simulink library "SimscapeFPGAHIL_lib"  (R2023b)
settings: Solver=VariableStepAuto  StartTime=0.0  StopTime=10.0  RelTol=1e-3
undefined symbols (not defined in the file): a, b, c, DiscIntNeverNeededParam, threshold
libraries: fl_lib x16, nesl_utility x12, simulink x10, fpga_utils_lib x4, hdlsllib x2, $bdroot x1
settings Model: Creator=The MathWorks, Inc.  LastModifiedBy=promero

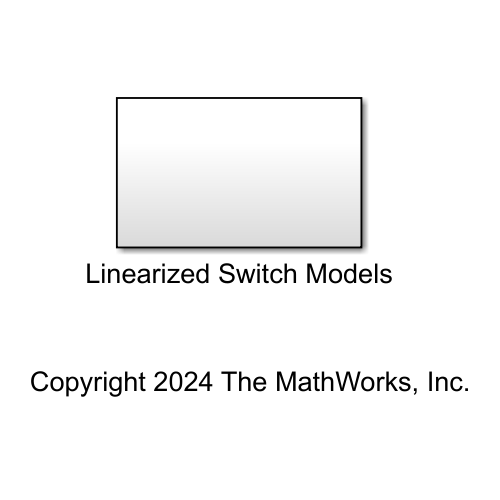
[thumbnail: Simulink's stored preview of the top-level diagram]
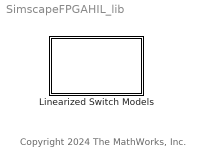
== system SimscapeFPGAHIL_lib ==
  note: Copyright 2024 The MathWorks, Inc.
  Linearized Switch Models : Subsystem

== system SimscapeFPGAHIL_lib/Linearized Switch Models ==
  note: Linear time-invariant approximation of piecewise linear switching elements
  Diode : Subsystem  mask{Vf=0.6, Gs=1, s=1}
      mask prompts: Vf "Forward voltage [V]"; Gs "Conductance (1/Ohm)"; s "Time scaling"
      settings: CopyFcn=set_param(gcb, 'LinkStatus', 'none');
      mask TypeOptions Vf: Controller/Vf
      mask TypeOptions s: Controller/s
  IGBT : Subsystem  mask{Vth=0.5, Vf=0.8, Gs=1, s=1, avgFactor=1, isFixedPoint=off}
      mask prompts: Vth "Threshold voltage [V]"; Vf "Forward voltage [V]"; Gs "Conductance [1/Ohm]"; s "Time scaling"; avgFactor "Subcycle average factor"; isFixedPoint "Use fixed point for Subcycle Average"
      settings: CopyFcn=set_param(gcb, 'LinkStatus', 'none');
      mask TypeOptions Vth: Controller/Vth
      mask TypeOptions Vf: Controller/Vf
      mask TypeOptions s: Controller/s
      mask TypeOptions avgFactor: Controller/avgFactor
      mask TypeOptions isFixedPoint: Controller/isFixedPoint
  MOSFET : Subsystem  mask{threshold=0.5, Gs=1, s=1, avgFactor=1, isFixedPoint=off}
      mask prompts: threshold "Threshold voltage [V]"; Gs "Conductance (1/Ohm)"; s "Time scaling"; avgFactor "Subcycle average factor"; isFixedPoint "Use fixed-point for Subcycle Average"
      settings: CopyFcn=set_param(gcb, 'LinkStatus', 'none');
      mask TypeOptions threshold: Controller/threshold
      mask TypeOptions s: Controller/s
      mask TypeOptions avgFactor: Controller/avgFactor
      mask TypeOptions isFixedPoint: Controller/isFixedPoint
  Switch : Subsystem  mask{threshold=0.5, Gs=1, s=1, avgFactor=1, isFixedPoint=off}
      mask prompts: threshold "Threshold voltage [V]"; Gs "Conductance (1/Ohm)"; s "Time scaling"; avgFactor "Subcycle average factor"; isFixedPoint "Use fixed-point for Subcycle Average"
      settings: CopyFcn=set_param(gcb, 'LinkStatus', 'none');
      mask TypeOptions threshold: Controller/threshold
      mask TypeOptions s: Controller/s
      mask TypeOptions avgFactor: Controller/avgFactor
      mask TypeOptions isFixedPoint: Controller/isFixedPoint

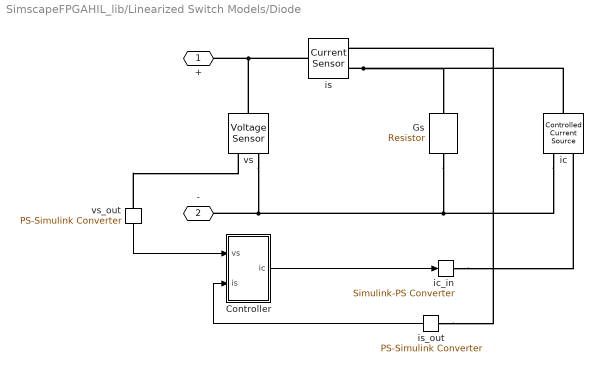
== system SimscapeFPGAHIL_lib/Linearized Switch Models/Diode ==
  Controller : Subsystem  mask{Vf=Vf, Gs=Gs, s=s}
      mask prompts: Vf "Forward voltage [V]"; Gs "Conductance [1/Ohm]"; s "Time scaling"
      mask DialogControl DescGroupVar Prompt: Description
      mask DialogControl Details Prompt: Diode Controller
  Gs : fl_lib/Electrical/Electrical Elements/Resistor  R=1/Gs Ohm  i_specify=off  i_priority=None  i=0 A  i_nominal_specify=off  i_nominal_unit=A  i_nominal_value=1  v_specify=off  v_priority=None  v=0 V  v_nominal_specify=off  v_nominal_unit=V  v_nominal_value=1
      settings: LibrarySourceBlock=SimscapeFPGAHIL_lib/Linearized Switch Models/Switch/Gs
  ic : fl_lib/Electrical/Electrical Sources/Controlled Current Source
      settings: LibrarySourceBlock=SimscapeFPGAHIL_lib/Linearized Switch Models/Switch/ic
  ic_in : nesl_utility/Simulink-PS Converter  PhysicalDomain=network_engine_domain  SubClassName=ps_input  LeftPortType=input  RightPortType=output  PseudoPeriodic=off  Frequencies=[]  NoiseDistribution=none  NoiseParameters=[]  Unit=A  AffineConversion=off  FilteringAndDerivatives=provide  SimscapeFilterOrder=1  InputFilterTimeConstant=0.001  UdotUserProvided=0
      settings: LibrarySourceBlock=SimscapeFPGAHIL_lib/Linearized Switch Models/Switch/ic_in
  is : fl_lib/Electrical/Electrical Sensors/Current Sensor
      settings: LibrarySourceBlock=SimscapeFPGAHIL_lib/Linearized Switch Models/Switch/is
  is_out : nesl_utility/PS-Simulink Converter  PhysicalDomain=network_engine_domain  SubClassName=ps_output  LeftPortType=input  RightPortType=output  PseudoPeriodic=off  Frequencies=[]  VectorFormat=1-D array  Unit=A  AffineConversion=off
      settings: LibrarySourceBlock=SimscapeFPGAHIL_lib/Linearized Switch Models/Switch/is_out
  vs : fl_lib/Electrical/Electrical Sensors/Voltage Sensor
      settings: LibrarySourceBlock=SimscapeFPGAHIL_lib/Linearized Switch Models/Switch/vs
  vs_out : nesl_utility/PS-Simulink Converter  PhysicalDomain=network_engine_domain  SubClassName=ps_output  LeftPortType=input  RightPortType=output  PseudoPeriodic=off  Frequencies=[]  VectorFormat=1-D array  Unit=V  AffineConversion=off
      settings: LibrarySourceBlock=SimscapeFPGAHIL_lib/Linearized Switch Models/Switch/vs_out
  + : PMIOPort  Side=Left
  - : PMIOPort  Port=2  Side=Right
  wires:
  Controller/1(ic) -> ic_in/1
  is_out/1 -> Controller/2(is)
  vs_out/1 -> Controller/1(vs)
  connections:
  is_out/LConn1 -- is/RConn1
  vs_out/LConn1 -- vs/RConn1
  ic_in/RConn1 -- ic/RConn1
  is/LConn1 -- +/RConn1 -- vs/LConn1
  ic/RConn2 -- Gs/RConn1 -- -/RConn1 -- vs/RConn2
  is/RConn2 -- Gs/LConn1 -- ic/LConn1

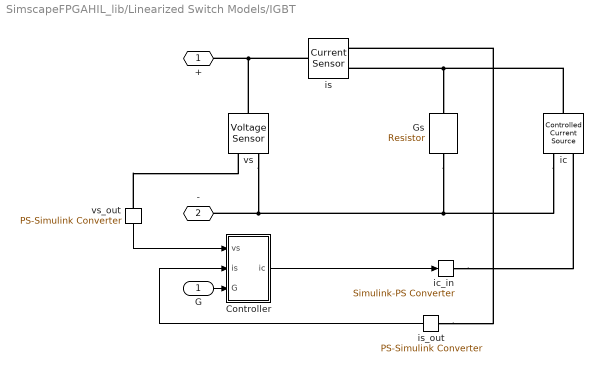
== system SimscapeFPGAHIL_lib/Linearized Switch Models/IGBT ==
  G : Inport
  Controller : Subsystem  mask{Vf=Vf, Vth=Vth, Gs=Gs, s=s, avgFactor=avgFactor, isFixedPoint=off}
      mask prompts: Vf "Forward voltage (V)"; Vth "Threshold voltage (V)"; Gs "Conductance (1/Ohm)"; s "Time scaling"; avgFactor "Subcycle average factor"; isFixedPoint "Use fixed point for Subcycle Average"
      mask DialogControl DescGroupVar Prompt: Description
      mask DialogControl Details Prompt: IGBT Controller
  Gs : fl_lib/Electrical/Electrical Elements/Resistor  R=1/Gs Ohm  i_specify=off  i_priority=None  i=0 A  i_nominal_specify=off  i_nominal_unit=A  i_nominal_value=1  v_specify=off  v_priority=None  v=0 V  v_nominal_specify=off  v_nominal_unit=V  v_nominal_value=1
      settings: LibrarySourceBlock=SimscapeFPGAHIL_lib/Linearized Switch Models/MOSFET/Gs
  ic : fl_lib/Electrical/Electrical Sources/Controlled Current Source
      settings: LibrarySourceBlock=SimscapeFPGAHIL_lib/Linearized Switch Models/MOSFET/ic
  ic_in : nesl_utility/Simulink-PS Converter  PhysicalDomain=network_engine_domain  SubClassName=ps_input  LeftPortType=input  RightPortType=output  PseudoPeriodic=off  Frequencies=[]  NoiseDistribution=none  NoiseParameters=[]  Unit=A  AffineConversion=off  FilteringAndDerivatives=provide  SimscapeFilterOrder=1  InputFilterTimeConstant=0.001  UdotUserProvided=0
      settings: LibrarySourceBlock=SimscapeFPGAHIL_lib/Linearized Switch Models/MOSFET/ic_in
  is : fl_lib/Electrical/Electrical Sensors/Current Sensor
      settings: LibrarySourceBlock=SimscapeFPGAHIL_lib/Linearized Switch Models/MOSFET/is
  is_out : nesl_utility/PS-Simulink Converter  PhysicalDomain=network_engine_domain  SubClassName=ps_output  LeftPortType=input  RightPortType=output  PseudoPeriodic=off  Frequencies=[]  VectorFormat=1-D array  Unit=A  AffineConversion=off
      settings: LibrarySourceBlock=SimscapeFPGAHIL_lib/Linearized Switch Models/MOSFET/is_out
  vs : fl_lib/Electrical/Electrical Sensors/Voltage Sensor
      settings: LibrarySourceBlock=SimscapeFPGAHIL_lib/Linearized Switch Models/MOSFET/vs
  vs_out : nesl_utility/PS-Simulink Converter  PhysicalDomain=network_engine_domain  SubClassName=ps_output  LeftPortType=input  RightPortType=output  PseudoPeriodic=off  Frequencies=[]  VectorFormat=1-D array  Unit=V  AffineConversion=off
      settings: LibrarySourceBlock=SimscapeFPGAHIL_lib/Linearized Switch Models/MOSFET/vs_out
  + : PMIOPort  Side=Left
  - : PMIOPort  Port=2  Side=Right
  wires:
  vs_out/1 -> Controller/1(vs)
  is_out/1 -> Controller/2(is)
  G/1 -> Controller/3(G)
  Controller/1(ic) -> ic_in/1
  connections:
  ic/LConn1 -- Gs/LConn1 -- is/RConn2
  vs/RConn2 -- -/RConn1 -- Gs/RConn1 -- ic/RConn2
  vs/LConn1 -- +/RConn1 -- is/LConn1
  ic_in/RConn1 -- ic/RConn1
  vs_out/LConn1 -- vs/RConn1
  is_out/LConn1 -- is/RConn1

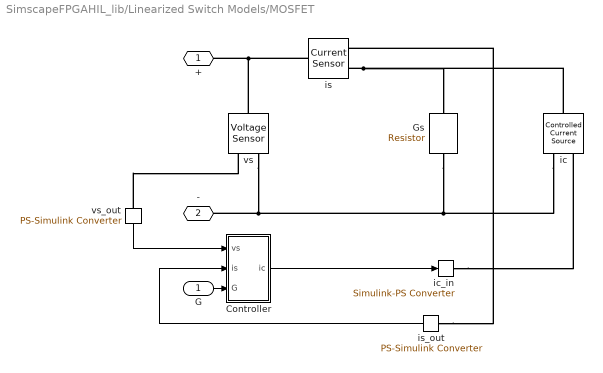
== system SimscapeFPGAHIL_lib/Linearized Switch Models/MOSFET ==
  G : Inport
  Controller : Subsystem  mask{threshold=threshold, Gs=Gs, s=s, avgFactor=avgFactor, isFixedPoint=off}
      mask prompts: threshold "Threshold voltage [V]"; Gs "Conductance (1/Ohm)"; s "Time scaling"; avgFactor "Subcycle average factor"; isFixedPoint "Use fixed-point for Subcycle Average"
      mask DialogControl DescGroupVar Prompt: Description
      mask DialogControl Details Prompt: Switch Controller
  Gs : fl_lib/Electrical/Electrical Elements/Resistor  R=1/Gs Ohm  i_specify=off  i_priority=None  i=0 A  i_nominal_specify=off  i_nominal_unit=A  i_nominal_value=1  v_specify=off  v_priority=None  v=0 V  v_nominal_specify=off  v_nominal_unit=V  v_nominal_value=1
  ic : fl_lib/Electrical/Electrical Sources/Controlled Current Source
  ic_in : nesl_utility/Simulink-PS Converter  PhysicalDomain=network_engine_domain  SubClassName=ps_input  LeftPortType=input  RightPortType=output  PseudoPeriodic=off  Frequencies=[]  NoiseDistribution=none  NoiseParameters=[]  Unit=A  AffineConversion=off  FilteringAndDerivatives=provide  SimscapeFilterOrder=1  InputFilterTimeConstant=0.001  UdotUserProvided=0
  is : fl_lib/Electrical/Electrical Sensors/Current Sensor
  is_out : nesl_utility/PS-Simulink Converter  PhysicalDomain=network_engine_domain  SubClassName=ps_output  LeftPortType=input  RightPortType=output  PseudoPeriodic=off  Frequencies=[]  VectorFormat=1-D array  Unit=A  AffineConversion=off
  vs : fl_lib/Electrical/Electrical Sensors/Voltage Sensor
  vs_out : nesl_utility/PS-Simulink Converter  PhysicalDomain=network_engine_domain  SubClassName=ps_output  LeftPortType=input  RightPortType=output  PseudoPeriodic=off  Frequencies=[]  VectorFormat=1-D array  Unit=V  AffineConversion=off
  + : PMIOPort  Side=Left
  - : PMIOPort  Port=2  Side=Right
  wires:
  Controller/1(ic) -> ic_in/1
  G/1 -> Controller/3(G)
  is_out/1 -> Controller/2(is)
  vs_out/1 -> Controller/1(vs)
  connections:
  is_out/LConn1 -- is/RConn1
  vs_out/LConn1 -- vs/RConn1
  ic_in/RConn1 -- ic/RConn1
  is/LConn1 -- +/RConn1 -- vs/LConn1
  ic/RConn2 -- Gs/RConn1 -- -/RConn1 -- vs/RConn2
  is/RConn2 -- Gs/LConn1 -- ic/LConn1

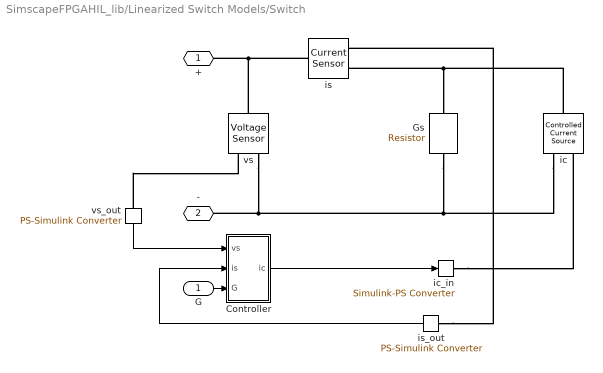
== system SimscapeFPGAHIL_lib/Linearized Switch Models/Switch ==
  G : Inport
  Controller : Subsystem  mask{threshold=threshold, Gs=Gs, s=s, avgFactor=avgFactor, isFixedPoint=off}
      mask prompts: threshold "Threshold voltage [V]"; Gs "Conductance (1/Ohm)"; s "Time scaling"; avgFactor "Subcycle average factor"; isFixedPoint "Use fixed-point for Subcycle Average"
      mask DialogControl DescGroupVar Prompt: Description
      mask DialogControl Details Prompt: Switch Controller
  Gs : fl_lib/Electrical/Electrical Elements/Resistor  R=1/Gs Ohm  i_specify=off  i_priority=None  i=0 A  i_nominal_specify=off  i_nominal_unit=A  i_nominal_value=1  v_specify=off  v_priority=None  v=0 V  v_nominal_specify=off  v_nominal_unit=V  v_nominal_value=1
  ic : fl_lib/Electrical/Electrical Sources/Controlled Current Source
  ic_in : nesl_utility/Simulink-PS Converter  PhysicalDomain=network_engine_domain  SubClassName=ps_input  LeftPortType=input  RightPortType=output  PseudoPeriodic=off  Frequencies=[]  NoiseDistribution=none  NoiseParameters=[]  Unit=A  AffineConversion=off  FilteringAndDerivatives=provide  SimscapeFilterOrder=1  InputFilterTimeConstant=0.001  UdotUserProvided=0
  is : fl_lib/Electrical/Electrical Sensors/Current Sensor
  is_out : nesl_utility/PS-Simulink Converter  PhysicalDomain=network_engine_domain  SubClassName=ps_output  LeftPortType=input  RightPortType=output  PseudoPeriodic=off  Frequencies=[]  VectorFormat=1-D array  Unit=A  AffineConversion=off
  vs : fl_lib/Electrical/Electrical Sensors/Voltage Sensor
  vs_out : nesl_utility/PS-Simulink Converter  PhysicalDomain=network_engine_domain  SubClassName=ps_output  LeftPortType=input  RightPortType=output  PseudoPeriodic=off  Frequencies=[]  VectorFormat=1-D array  Unit=V  AffineConversion=off
  + : PMIOPort  Side=Left
  - : PMIOPort  Port=2  Side=Right
  wires:
  vs_out/1 -> Controller/1(vs)
  is_out/1 -> Controller/2(is)
  G/1 -> Controller/3(G)
  Controller/1(ic) -> ic_in/1
  connections:
  ic/LConn1 -- Gs/LConn1 -- is/RConn2
  vs/RConn2 -- -/RConn1 -- Gs/RConn1 -- ic/RConn2
  vs/LConn1 -- +/RConn1 -- is/LConn1
  ic_in/RConn1 -- ic/RConn1
  vs_out/LConn1 -- vs/RConn1
  is_out/LConn1 -- is/RConn1

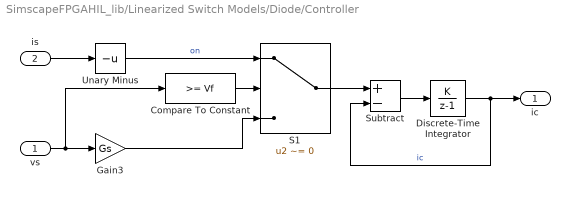
== system SimscapeFPGAHIL_lib/Linearized Switch Models/Diode/Controller ==
  vs : Inport
  is : Inport  Port=2
  Compare To Constant : simulink/Logic and Bit Operations/Compare To Constant  relop=>=  const=Vf  OutDataTypeStr=boolean
      settings: LibrarySourceBlock=|
      | SimscapeFPGAHIL_lib/Linearized Switch Models/Switch/Controller/Switch State/Switch/Compare
      | To Constant
  Discrete-Time Integrator : DiscreteIntegrator  IntegratorMethod=Accumulation: Forward Euler  gainval=1/s  SampleTime=-1  OutDataTypeStr=Inherit: Inherit via back propagation  ICPrevOutput=DiscIntNeverNeededParam  ICPrevScaledInput=DiscIntNeverNeededParam
  Gain3 : Gain  Gain=Gs  OutDataTypeStr=Inherit: Inherit via back propagation
  S1 : Switch  Criteria=u2 ~= 0  Threshold=threshold  SaturateOnIntegerOverflow=off
  Subtract : Sum  Inputs=+-
  Unary Minus : UnaryMinus
  ic : Outport
  wires:
  vs/1 -> Compare To Constant/1, Gain3/1
  is/1 -> Unary Minus/1
  Discrete-Time Integrator/1 -> ic/1, Subtract/2  "ic"
  Subtract/1 -> Discrete-Time Integrator/1
  Gain3/1 -> S1/3
  Unary Minus/1 -> S1/1  "on"
  Compare To Constant/1 -> S1/2
  S1/1 -> Subtract/1

== system SimscapeFPGAHIL_lib/Linearized Switch Models/IGBT/Controller ==
  vs : Inport
  is : Inport  Port=2
  G : Inport  Port=3
  Discrete-Time Integrator : DiscreteIntegrator  IntegratorMethod=Accumulation: Forward Euler  gainval=1/s  SampleTime=-1  OutDataTypeStr=Inherit: Inherit via back propagation  ICPrevOutput=DiscIntNeverNeededParam  ICPrevScaledInput=DiscIntNeverNeededParam
  Subtract : Sum  Inputs=+-
  Switch State : Subsystem  Variant=on  VariantControl=Choice
  Unary Minus : UnaryMinus
  ic : Outport
  wires:
  Unary Minus/1 -> Switch State/1(on)  "on"
  Switch State/1(ic) -> Subtract/1
  Subtract/1 -> Discrete-Time Integrator/1
  Discrete-Time Integrator/1 -> Subtract/2, ic/1  "ic"
  is/1 -> Unary Minus/1
  vs/1 -> Switch State/3(vs)
  G/1 -> Switch State/2(G)

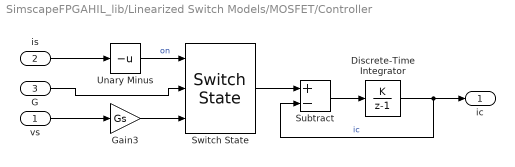
== system SimscapeFPGAHIL_lib/Linearized Switch Models/MOSFET/Controller ==
  vs : Inport
  is : Inport  Port=2
  G : Inport  Port=3
  Discrete-Time Integrator : DiscreteIntegrator  IntegratorMethod=Accumulation: Forward Euler  gainval=1/s  SampleTime=-1  OutDataTypeStr=Inherit: Inherit via back propagation  ICPrevOutput=DiscIntNeverNeededParam  ICPrevScaledInput=DiscIntNeverNeededParam
  Gain3 : Gain  Gain=Gs  OutDataTypeStr=Inherit: Inherit via back propagation
  Subtract : Sum  Inputs=+-
  Switch State : $bdroot/Linearized Switch Models/Switch/Controller/Switch State  SystemSampleTime=-1  VariantControl=Choice  VariantActivationTime=update diagram  AllowFlexibleInterface=on  Latency=0  AutoFrameSizeCalculation=off
      settings: LibrarySourceBlock=SimscapeFPGAHIL_lib/Linearized Switch Models/MOSFET/Controller/Controller/Switch State
  Unary Minus : UnaryMinus
  ic : Outport
  wires:
  Switch State/1 -> Subtract/1
  Gain3/1 -> Switch State/3
  G/1 -> Switch State/2
  Unary Minus/1 -> Switch State/1  "on"
  is/1 -> Unary Minus/1
  Discrete-Time Integrator/1 -> ic/1, Subtract/2  "ic"
  Subtract/1 -> Discrete-Time Integrator/1
  vs/1 -> Gain3/1

== system SimscapeFPGAHIL_lib/Linearized Switch Models/Switch/Controller ==
  vs : Inport
  is : Inport  Port=2
  G : Inport  Port=3
  Discrete-Time Integrator : DiscreteIntegrator  IntegratorMethod=Accumulation: Forward Euler  gainval=1/s  SampleTime=-1  OutDataTypeStr=Inherit: Inherit via back propagation  ICPrevOutput=DiscIntNeverNeededParam  ICPrevScaledInput=DiscIntNeverNeededParam
  Gain3 : Gain  Gain=Gs  OutDataTypeStr=Inherit: Inherit via back propagation
  Subtract : Sum  Inputs=+-
  Switch State : Subsystem  Variant=on  VariantControl=Choice
  Unary Minus : UnaryMinus
  ic : Outport
  wires:
  vs/1 -> Gain3/1
  Subtract/1 -> Discrete-Time Integrator/1
  Discrete-Time Integrator/1 -> ic/1, Subtract/2  "ic"
  is/1 -> Unary Minus/1
  Unary Minus/1 -> Switch State/1(on)  "on"
  G/1 -> Switch State/2(G)
  Gain3/1 -> Switch State/3(off)
  Switch State/1(ic) -> Subtract/1

== system SimscapeFPGAHIL_lib/Linearized Switch Models/IGBT/Controller/Switch State ==
  on : Inport
  G : Inport  Port=2
  vs : Inport  Port=3
  Subcycle Average (Fixed Point) : Subsystem  VariantControl=avgFactor > 1 && isFixedPoint
      settings: LibrarySourceBlock=SimscapeFPGAHIL_lib/Linearized Switch Models/IGBT/Controller/Switch State/Subcycle Average
  Subcycle Average (Floating Point) : Subsystem  VariantControl=avgFactor > 1 && ~isFixedPoint
  Switch : Subsystem  VariantControl=avgFactor == 1
  ic : Outport

== system SimscapeFPGAHIL_lib/Linearized Switch Models/Switch/Controller/Switch State ==
  on : Inport
  G : Inport  Port=2
  off : Inport  Port=3
  Subcycle Average (Fixed-Point) : Subsystem  VariantControl=avgFactor > 1 && isFixedPoint == true
  Subcycle Average (Floating-Point) : Subsystem  VariantControl=avgFactor > 1 && isFixedPoint == false
  Switch : Subsystem  VariantControl=avgFactor == 1
  ic : Outport

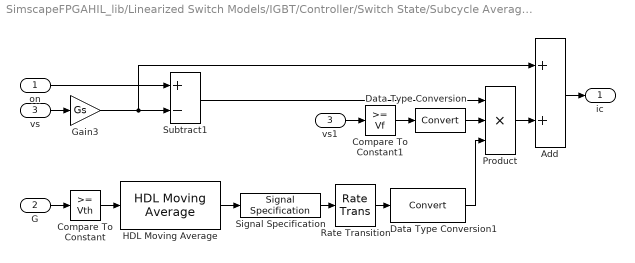
== system SimscapeFPGAHIL_lib/Linearized Switch Models/IGBT/Controller/Switch State/Subcycle Average (Fixed Point) ==
  on : Inport
  G : Inport  Port=2
  vs : Inport  Port=3
  Add : Sum
  Compare To Constant : simulink/Logic and Bit Operations/Compare To Constant  relop=>=  const=Vth  OutDataTypeStr=boolean
      settings: LibrarySourceBlock=|
      | SimscapeFPGAHIL_lib/Linearized Switch Models/IGBT/Controller/Switch State/Subcycle Average/Compare
      | To Constant
  Compare To Constant1 : simulink/Logic and Bit Operations/Compare To Constant  relop=>=  const=Vf  OutDataTypeStr=boolean
      settings: LibrarySourceBlock=|
      | SimscapeFPGAHIL_lib/Linearized Switch Models/IGBT/Controller/Switch State/Subcycle Average/Compare
      | To Constant1
  Data Type Conversion : DataTypeConversion  SaturateOnIntegerOverflow=off  RndMeth=Floor
  Data Type Conversion1 : DataTypeConversion  SaturateOnIntegerOverflow=off  RndMeth=Floor
  Gain3 : Gain  Gain=Gs
  HDL Moving Average : fpga_utils_lib/HDL Moving Average  avgRatio=avgFactor
  Product : Product  Inputs=3  InputSameDT=on
  Rate Transition : RateTransition  OutPortSampleTimeOpt=Multiple of input port sample time  OutPortSampleTimeMultiple=avgFactor
  Signal Specification : SignalSpecification  OutMin=0  OutMax=1  OutDataTypeStr=fixdt(0,15,14)
      settings: LockScale=on
  Subtract1 : Sum  Inputs=+-
  vs1 : InportShadow  Port=3
  ic : Outport
  wires:
  Data Type Conversion/1 -> Product/2
  Compare To Constant1/1 -> Data Type Conversion/1
  vs1/1 -> Compare To Constant1/1
  Product/1 -> Add/2
  Gain3/1 -> Subtract1/2, Add/1
  Add/1 -> ic/1
  Subtract1/1 -> Product/1
  Compare To Constant/1 -> HDL Moving Average/1
  G/1 -> Compare To Constant/1
  vs/1 -> Gain3/1
  on/1 -> Subtract1/1
  Signal Specification/1 -> Rate Transition/1
  Rate Transition/1 -> Data Type Conversion1/1
  Data Type Conversion1/1 -> Product/3
  HDL Moving Average/1 -> Signal Specification/1

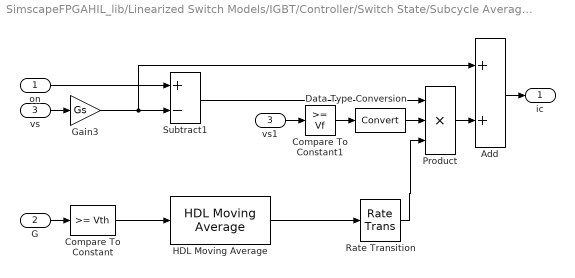
== system SimscapeFPGAHIL_lib/Linearized Switch Models/IGBT/Controller/Switch State/Subcycle Average (Floating Point) ==
  on : Inport
  G : Inport  Port=2
  vs : Inport  Port=3
  Add : Sum
  Compare To Constant : simulink/Logic and Bit Operations/Compare To Constant  relop=>=  const=Vth  OutDataTypeStr=boolean
  Compare To Constant1 : simulink/Logic and Bit Operations/Compare To Constant  relop=>=  const=Vf  OutDataTypeStr=boolean
  Data Type Conversion : DataTypeConversion  SaturateOnIntegerOverflow=off  RndMeth=Floor
  Gain3 : Gain  Gain=Gs
  HDL Moving Average : fpga_utils_lib/HDL Moving Average  avgRatio=avgFactor
  Product : Product  Inputs=3  InputSameDT=on
  Rate Transition : RateTransition  OutPortSampleTimeOpt=Multiple of input port sample time  OutPortSampleTimeMultiple=avgFactor
  Subtract1 : Sum  Inputs=+-  OutDataTypeStr=Inherit: Same as first input
  vs1 : InportShadow  Port=3
  ic : Outport
  wires:
  on/1 -> Subtract1/1
  vs/1 -> Gain3/1
  G/1 -> Compare To Constant/1
  Compare To Constant/1 -> HDL Moving Average/1
  Subtract1/1 -> Product/1
  Add/1 -> ic/1
  Gain3/1 -> Add/1, Subtract1/2
  Product/1 -> Add/2
  vs1/1 -> Compare To Constant1/1
  Compare To Constant1/1 -> Data Type Conversion/1
  Rate Transition/1 -> Product/3
  Data Type Conversion/1 -> Product/2
  HDL Moving Average/1 -> Rate Transition/1

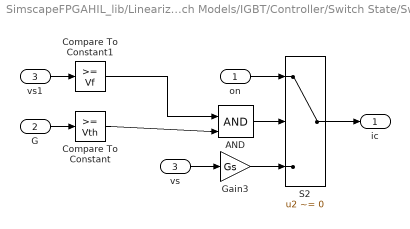
== system SimscapeFPGAHIL_lib/Linearized Switch Models/IGBT/Controller/Switch State/Switch ==
  on : Inport
  G : Inport  Port=2
  vs : Inport  Port=3
  AND : Logic  IconShape=distinctive  AllPortsSameDT=off  OutDataTypeStr=boolean
  Compare To Constant : simulink/Logic and Bit Operations/Compare To Constant  relop=>=  const=Vth  OutDataTypeStr=boolean
      settings: LibrarySourceBlock=|
      | SimscapeFPGAHIL_lib/Linearized Switch Models/Controller/Switch State/Switch/Compare
      | To Constant
  Compare To Constant1 : simulink/Logic and Bit Operations/Compare To Constant  relop=>=  const=Vf  OutDataTypeStr=boolean
      settings: LibrarySourceBlock=|
      | SimscapeFPGAHIL_lib/Linearized Switch Models/Controller/Switch State/Switch/Compare
      | To Constant1
  Gain3 : Gain  Gain=Gs  OutDataTypeStr=Inherit: Inherit via back propagation
  S2 : Switch  Criteria=u2 ~= 0  Threshold=threshold  SaturateOnIntegerOverflow=off
  vs1 : InportShadow  Port=3
  ic : Outport
  wires:
  on/1 -> S2/1
  S2/1 -> ic/1
  vs/1 -> Gain3/1
  Gain3/1 -> S2/3
  Compare To Constant1/1 -> AND/1
  Compare To Constant/1 -> AND/2
  AND/1 -> S2/2
  G/1 -> Compare To Constant/1
  vs1/1 -> Compare To Constant1/1

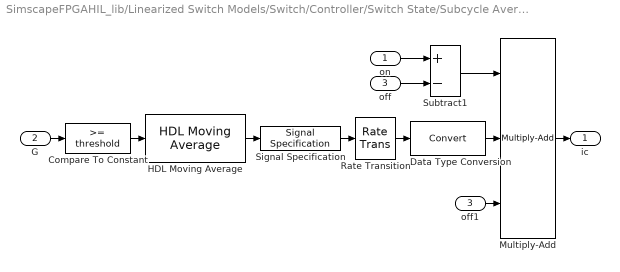
== system SimscapeFPGAHIL_lib/Linearized Switch Models/Switch/Controller/Switch State/Subcycle Average (Fixed-Point) ==
  on : Inport
  G : Inport  Port=2
  off : Inport  Port=3
  Compare To Constant : simulink/Logic and Bit Operations/Compare To Constant  relop=>=  const=threshold  OutDataTypeStr=boolean
  Data Type Conversion : DataTypeConversion  SaturateOnIntegerOverflow=off  RndMeth=Floor
  HDL Moving Average : fpga_utils_lib/HDL Moving Average  avgRatio=avgFactor
  Multiply-Add : hdlsllib/HDL Operations/Multiply-Add  Function=c+(a.*b)  datatype=Inherit: Inherit via internal rule  DoSatur=off  FMA=off
      settings: LibrarySourceBlock=SimscapeFPGAHIL_lib/Linearized Switch Models/Switch/Controller/Switch State/Subcycle Average (Floating-Point)/Multiply-Add
  Rate Transition : RateTransition  OutPortSampleTimeOpt=Multiple of input port sample time  OutPortSampleTimeMultiple=avgFactor
  Signal Specification : SignalSpecification  OutMin=0  OutMax=1  OutDataTypeStr=fixdt(0,15,14)
      settings: LockScale=on
  Subtract1 : Sum  Inputs=+-
  off1 : InportShadow  Port=3
  ic : Outport
  wires:
  Data Type Conversion/1 -> Multiply-Add/2
  Signal Specification/1 -> Rate Transition/1
  Rate Transition/1 -> Data Type Conversion/1
  Subtract1/1 -> Multiply-Add/1
  G/1 -> Compare To Constant/1
  off/1 -> Subtract1/2
  on/1 -> Subtract1/1
  Compare To Constant/1 -> HDL Moving Average/1
  HDL Moving Average/1 -> Signal Specification/1
  off1/1 -> Multiply-Add/3
  Multiply-Add/1 -> ic/1

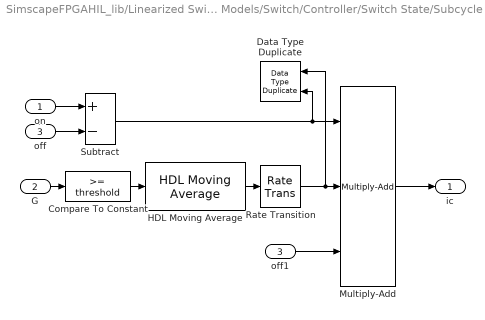
== system SimscapeFPGAHIL_lib/Linearized Switch Models/Switch/Controller/Switch State/Subcycle Average (Floating-Point) ==
  on : Inport
  G : Inport  Port=2
  off : Inport  Port=3
  Compare To Constant : simulink/Logic and Bit Operations/Compare To Constant  relop=>=  const=threshold  OutDataTypeStr=boolean
  Data Type Duplicate : DataTypeDuplicate
  HDL Moving Average : fpga_utils_lib/HDL Moving Average  avgRatio=avgFactor
  Multiply-Add : hdlsllib/HDL Operations/Multiply-Add  Function=c+(a.*b)  datatype=Inherit: Inherit via internal rule  DoSatur=off  FMA=off
  Rate Transition : RateTransition  OutPortSampleTimeOpt=Multiple of input port sample time  OutPortSampleTimeMultiple=avgFactor
  Subtract : Sum  Inputs=+-  OutDataTypeStr=Inherit: Same as first input
  off1 : InportShadow  Port=3
  ic : Outport
  wires:
  on/1 -> Subtract/1
  off/1 -> Subtract/2
  G/1 -> Compare To Constant/1
  Compare To Constant/1 -> HDL Moving Average/1
  Subtract/1 -> Data Type Duplicate/2, Multiply-Add/1
  Rate Transition/1 -> Data Type Duplicate/1, Multiply-Add/2
  HDL Moving Average/1 -> Rate Transition/1
  off1/1 -> Multiply-Add/3
  Multiply-Add/1 -> ic/1

== system SimscapeFPGAHIL_lib/Linearized Switch Models/Switch/Controller/Switch State/Switch ==
  on : Inport
  G : Inport  Port=2
  off : Inport  Port=3
  Compare To Constant : simulink/Logic and Bit Operations/Compare To Constant  relop=>=  const=threshold  OutDataTypeStr=boolean
      settings: LibrarySourceBlock=|
      | SimscapeFPGAHIL_lib/Linearized Switch Models/Switch/Controller/Switch State/Switch/Compare
      | To Constant
  S2 : Switch  Criteria=u2 ~= 0  Threshold=threshold  SaturateOnIntegerOverflow=off
  ic : Outport
  wires:
  on/1 -> S2/1
  S2/1 -> ic/1
  G/1 -> Compare To Constant/1
  off/1 -> S2/3
  Compare To Constant/1 -> S2/2
